simulink model "vidu_1"  (R2021a)
settings: Solver=VariableStepAuto  StartTime=0.0  StopTime=10.0  RelTol=1e-3
settings Model: Creator=HanO  LastModifiedBy=HanO

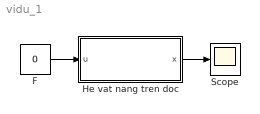
== system vidu_1 ==
  F : Constant  Value=0
  He vat nang tren doc : Subsystem  mask{m=3, g=9.81, alpha=pi/6, x0=0}
      mask prompts: m "Khối lượng vật nặng m [kg]"; g "Gia tốc trọng trường [m/s2]"; alpha "Độ nghiêng của dốc [rad]"; x0 "Vị trí đầu của vật nặng"
  Scope : Scope
  wires:
  He vat nang tren doc/1(x) -> Scope/1
  F/1 -> He vat nang tren doc/1(u)

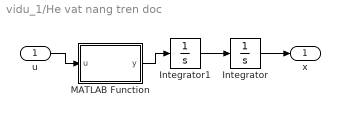
== system vidu_1/He vat nang tren doc ==
  u : Inport
  Integrator : Integrator  InitialCondition=x0
  Integrator1 : Integrator
  MATLAB Function : MATLAB Function  TreatAsAtomicUnit=on
  x : Outport
  wires:
  Integrator/1 -> x/1
  Integrator1/1 -> Integrator/1
  MATLAB Function/1(y) -> Integrator1/1
  u/1 -> MATLAB Function/1(u)

== matlab function vidu_1/He vat nang tren doc/MATLAB Function ==
  data: u input; y output
function y = fcn(u)
y = (u-m*g*sin(alpha))/m;
